simulink model "examp2"  (Simulink 4.00)
settings: Solver=ode45  StartTime=0.0  StopTime=10.0  RelTol=1e-3
settings Model: LastModifiedBy=User

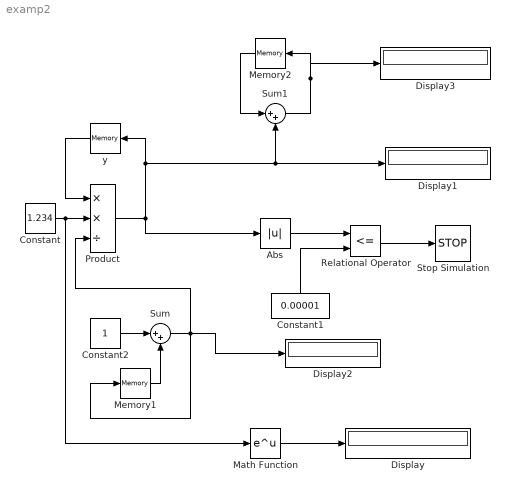
== system examp2 ==
  Abs : Abs  SaturateOnIntegerOverflow=on
  Constant : Constant  Value=1.234
  Constant1 : Constant  Orientation=up  Value=0.00001
  Constant2 : Constant  Value=1
  Display{,1..3} (4 alike) : Display
      Display2 settings: Format=short
  Math Function : Math  Operator=exp  OutputSignalType=auto
  Memory1 : Memory  X0=0  InheritSampleTime=off
      settings: RTWStateStorageClass=Auto
  Memory2 : Memory  Orientation=left  X0=1  InheritSampleTime=off
      settings: RTWStateStorageClass=Auto
  Product : Product  Inputs=**/  Multiplication=Element-wise(.*)  SaturateOnIntegerOverflow=off
  Relational Operator : RelationalOperator  Operator=<=
  Stop Simulation : Stop
  Sum : Sum  Inputs=|++  SaturateOnIntegerOverflow=on
  Sum1 : Sum  Inputs=|++  SaturateOnIntegerOverflow=off
  y : Memory  Orientation=left  X0=1  InheritSampleTime=off
      settings: RTWStateStorageClass=Auto
  wires:
  Constant/1 -> Product/2, Math Function/1
  Math Function/1 -> Display/1
  y/1 -> Product/1
  Product/1 -> y/1, Display1/1, Sum1/2, Abs/1
  Abs/1 -> Relational Operator/1
  Constant1/1 -> Relational Operator/2
  Relational Operator/1 -> Stop Simulation/1
  Constant2/1 -> Sum/1
  Memory1/1 -> Sum/2
  Sum/1 -> Memory1/1, Product/3, Display2/1
  Sum1/1 -> Memory2/1, Display3/1
  Memory2/1 -> Sum1/1
